simulink model "SIMMRACDISCRETO"  (R2022a)
settings: Solver=VariableStepAuto  StartTime=0.0  StopTime=10  RelTol=1e-3
values from neighbouring files (symbols this model uses):
  f = zeros(2*n,1)    [LAB.m]    (also in MRACdiscretoLab2.m = [(nd2*1)/(b1) 0])
  polinomioP = conv(bp, psol)    [MRACdiscretoLab2.m]
  T = 0.001    [GananciaProgramadaLab2.m]    (also in MRACdiscretoLab2.m = 0.470737468013)
undefined symbols (not defined in the file or in its folder): dd, nd, qsol
settings Model: Creator=salas  LastModifiedBy=PERSONAL

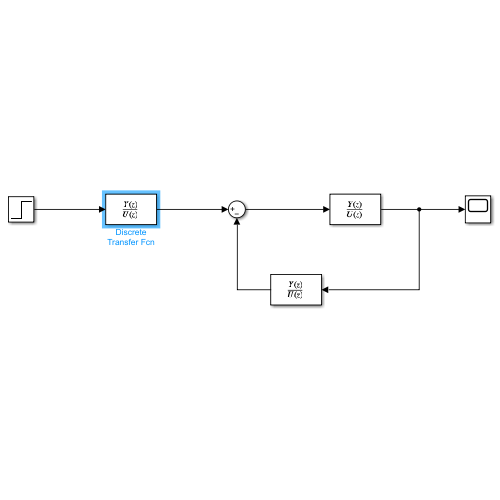
[thumbnail: Simulink's stored preview of the top-level diagram]
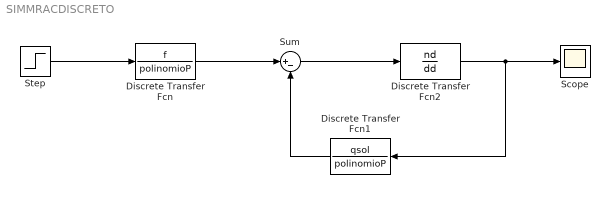
== system SIMMRACDISCRETO ==
  Discrete Transfer Fcn : DiscreteTransferFcn  Numerator=f  Denominator=polinomioP  SampleTime=T
  Discrete Transfer Fcn1 : DiscreteTransferFcn  Numerator=qsol  Denominator=polinomioP  SampleTime=T
  Discrete Transfer Fcn2 : DiscreteTransferFcn  Numerator=nd  Denominator=dd  SampleTime=T
  Scope : Scope
  Step : Step  Time=0  SampleTime=0
  Sum : Sum  Inputs=|+-
  wires:
  Step/1 -> Discrete Transfer Fcn/1
  Discrete Transfer Fcn/1 -> Sum/1
  Discrete Transfer Fcn1/1 -> Sum/2
  Discrete Transfer Fcn2/1 -> Discrete Transfer Fcn1/1, Scope/1
  Sum/1 -> Discrete Transfer Fcn2/1
